simulink model "EEG_Acquire_Works"  (R2014a)
settings: Solver=FixedStepDiscrete  StartTime=0.0  StopTime=600  FixedStep=1/250  MaxStep=1/250  RelTol=1e-3
InitFcn:
  | clear global handle
  | 
  | clear global userData
settings Model: Creator=ankit  LastModifiedBy=Sun Han
settings SolverCC: AutoInsertRateTranBlk=on  InsertRTBMode=Always
settings DataIOCC: LimitDataPoints=off  SignalLoggingSaveFormat=ModelDataLogs
settings OptimizationCC: ExpressionDepthLimit=2147483647  InitFltsAndDblsToZero=on
settings DebuggingCC: SaveWithParameterizedLinksMsg=none  UnderspecifiedInitializationDetection=Classic  SignalResolutionControl=TryResolveAllWithWarning  MultiTaskDSMMsg=warning  MultiTaskCondExecSysMsg=none  FcnCallInpInsideContextMsg=UseLocalSettings  StateNameClashWarn=warning
settings RTWCC: IncludeERTFirstTime=on
settings GRTTargetCC: TargetFcnLib=ansi_tfl_tmw.mat  CombineOutputUpdateFcns=off  GRTInterface=on

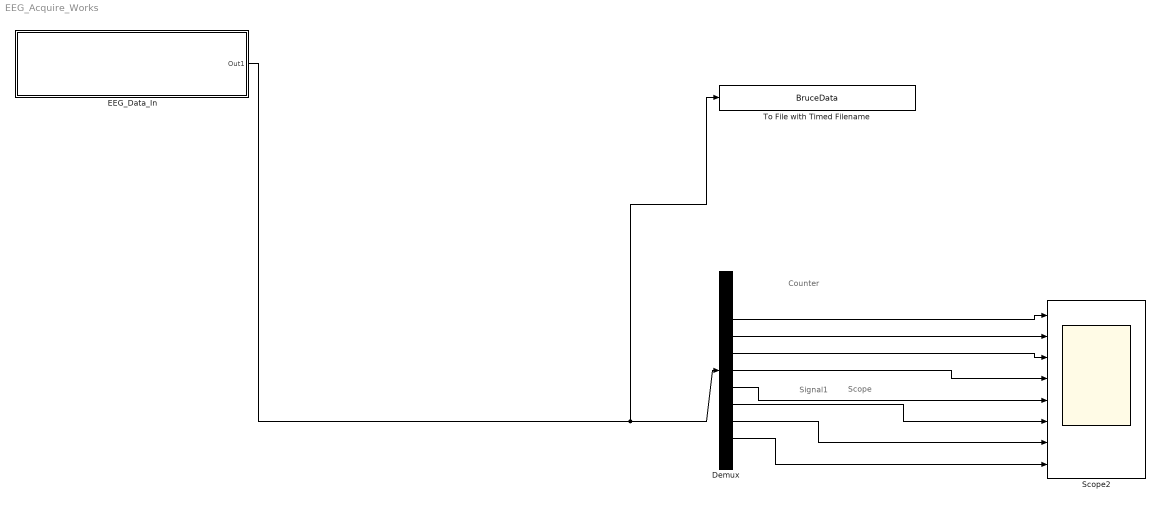
== system EEG_Acquire_Works ==
  note: Scope
  note: Counter
  note: Signal1
  Demux : Demux  Outputs=11
  EEG_Data_In : Subsystem  mask{COMPort=COM42, SPS=250}
      mask prompts: COMPort "COM Port"
      mask TypeOptions COMPort: COM1 | COM2 | COM3 | COM4 | COM5 | COM6 | COM7 | COM8 | COM9 | COM10 | COM11 | COM42 | COM13 | COM14 | COM15 | COM16 | COM17 | COM18 | COM19 | COM20 | COM21 | COM22 | COM23 | COM24 | COM25 | COM26 | COM27 | COM28 | COM29 | COM30 | COM31 | COM32
      mask TypeOptions SPS: 250 | 500 | 1000 | 2000 | 4000
      mask Display: port_label('output',1,'Data')
  Scope2 : Scope  NumInputPorts=8
      settings: ShowLegends=on  TimeRange=10  YMin=-8675~-29425~-44400~1900~-11300~-9450~1050~-2025  YMax=-8500~-29225~-44125~2100~-10950~-9150~1250~-1850  MaxDataPoints=50000  SampleInput=on
  To File with Timed Filename : ToFile  InitFcn=|  StopFcn=|  Filename=BruceData  MatrixName=y
      InitFcn=|
      | time=clock;                                                                                                                                                        
      | filenameToFilebase =  get_param(gcb,'Filename');                                                                                                                   
      | rename = [filenameToFilebase '_' num2str(time(1)) '_' num2str(time(2)) '_' num2str(time(3)) '_' num2str(time(4)) '_' num2str(time(5)) '_' num2str(round(time(6)))];
      | set_param(gcb,'Filename',rename);                                 clear time;                                                       clear rename;
      StopFcn=|
      | set_param(gcb,'Filename',filenameToFilebase);
      |                                              
      | clear filenameToFilebase
      settings: AttributesFormatString=Enter Base name, time will be added
  wires:
  EEG_Data_In/1(Out1) -> Demux/1, To File with Timed Filename/1
  Demux/3 -> Scope2/1
  Demux/4 -> Scope2/2
  Demux/5 -> Scope2/3
  Demux/6 -> Scope2/4
  Demux/7 -> Scope2/5
  Demux/8 -> Scope2/6
  Demux/9 -> Scope2/7
  Demux/10 -> Scope2/8

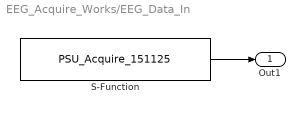
== system EEG_Acquire_Works/EEG_Data_In ==
  S-Function : S-Function  FunctionName=PSU_Acquire_151125  Parameters=COMPort,SPS  EnableBusSupport=off
  Out1 : Outport
  wires:
  S-Function/1 -> Out1/1
